simulink model "force_control_inner_loop"  (R2023a)
settings: Solver=VariableStepAuto  StartTime=0.0  StopTime=4  RelTol=1e-3
undefined symbols (not defined in the file): dqi, fd, invMd, K, KD, KF, KI, KP, Md, qi, robot, xr
settings Model: Creator=franc  LastModifiedBy=franc

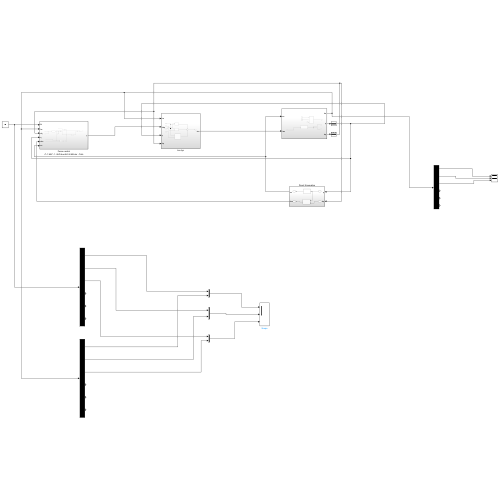
[thumbnail: Simulink's stored preview of the top-level diagram]
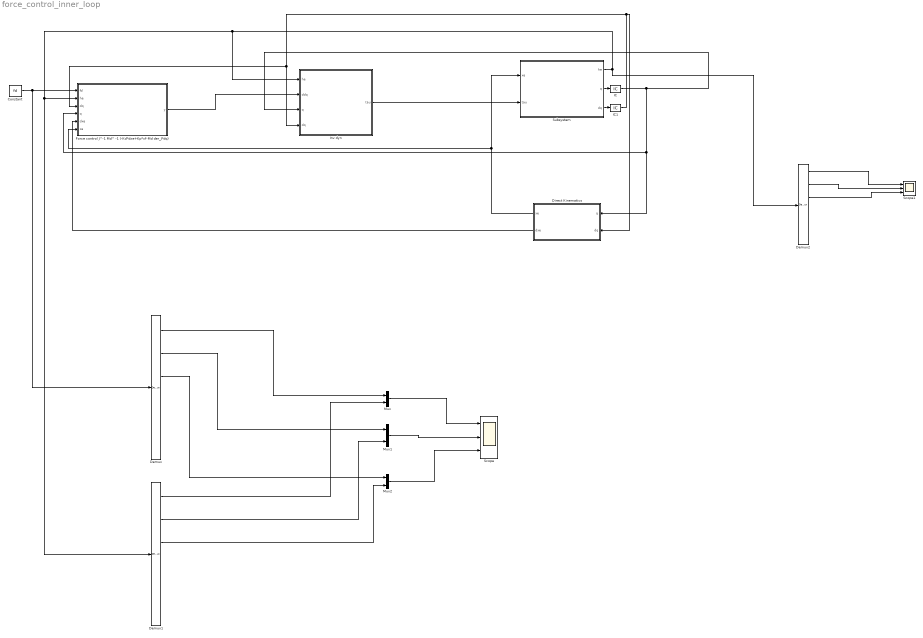
== system force_control_inner_loop ==
  Constant : Constant  Value=fd
  Demux : Demux  Outputs=6
  Demux1 : Demux  Outputs=6
  Demux2 : Demux  Outputs=6
  Direct Kinematics : Subsystem
  Force control J^-1 Md^ -1 (-Kd*dxe+Kp*xf-Md der_J*dq) : Subsystem
  IC : InitialCondition  Value=[0 0 0]
  IC1 : InitialCondition  Value=[0 0 0]
  Inv dyn : Subsystem
  Mux : Mux  Inputs=2
  Mux1 : Mux  Inputs=2
  Mux2 : Mux  Inputs=2
  Scope : Scope  NumInputPorts=3
  Scope1 : Scope  NumInputPorts=3
  Subsystem : Subsystem
  wires:
  Inv dyn/1(tau) -> Subsystem/2(tau)
  Subsystem/2(q) -> IC/1
  Subsystem/3(dq) -> IC1/1
  Direct Kinematics/1(xe) -> Subsystem/1(xe), Force control J^-1 Md^ -1 (-Kd*dxe+Kp*xf-Md der_J*dq)/6(xe)
  Direct Kinematics/2(dxe) -> Force control J^-1 Md^ -1 (-Kd*dxe+Kp*xf-Md der_J*dq)/5(dxe)
  Subsystem/1(he) -> Demux2/1, Inv dyn/1(he), Demux1/1, Force control J^-1 Md^ -1 (-Kd*dxe+Kp*xf-Md der_J*dq)/2(he)
  Force control J^-1 Md^ -1 (-Kd*dxe+Kp*xf-Md der_J*dq)/1(y) -> Inv dyn/2(ddq)
  Constant/1 -> Force control J^-1 Md^ -1 (-Kd*dxe+Kp*xf-Md der_J*dq)/1(fd), Demux/1
  Demux/1 -> Mux/1
  Demux/2 -> Mux1/1
  Demux/3 -> Mux2/1
  Demux1/1 -> Mux/2
  Demux1/2 -> Mux1/2
  Demux1/3 -> Mux2/2
  Mux/1 -> Scope/1
  Mux1/1 -> Scope/2
  Mux2/1 -> Scope/3
  IC/1 -> Force control J^-1 Md^ -1 (-Kd*dxe+Kp*xf-Md der_J*dq)/4(q), Direct Kinematics/1(q), Inv dyn/3(q)
  IC1/1 -> Force control J^-1 Md^ -1 (-Kd*dxe+Kp*xf-Md der_J*dq)/3(dq), Inv dyn/4(dq), Direct Kinematics/2(dq)
  Demux2/2 -> Scope1/2
  Demux2/1 -> Scope1/1
  Demux2/3 -> Scope1/3

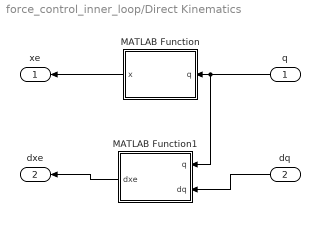
== system force_control_inner_loop/Direct Kinematics ==
  q : Inport
  dq : Inport  Port=2
  MATLAB Function : MATLAB Function  TreatAsAtomicUnit=on
  MATLAB Function1 : MATLAB Function  TreatAsAtomicUnit=on
  xe : Outport
  dxe : Outport  Port=2
  wires:
  dq/1 -> MATLAB Function1/2(dq)
  MATLAB Function1/1(dxe) -> dxe/1
  MATLAB Function/1(x) -> xe/1
  q/1 -> MATLAB Function/1(q), MATLAB Function1/1(q)

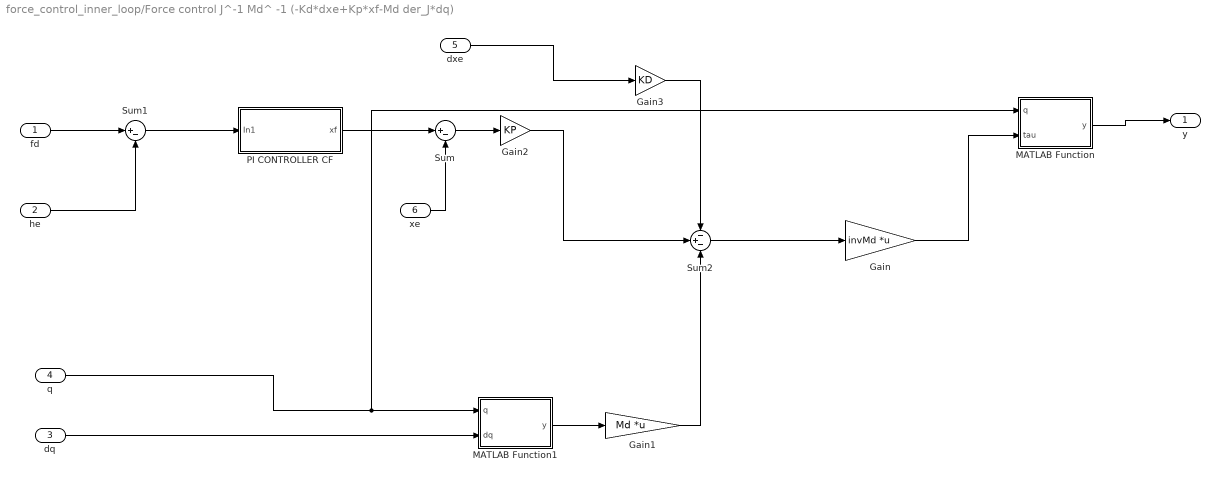
== system force_control_inner_loop/Force control J^-1 Md^ -1 (-Kd*dxe+Kp*xf-Md der_J*dq) ==
  fd : Inport
  he : Inport  Port=2
  dq : Inport  Port=3
  q : Inport  Port=4
  dxe : Inport  Port=5
  xe : Inport  Port=6
  Gain : Gain  Gain=invMd  Multiplication=Matrix(K*u)
  Gain1 : Gain  Gain=Md  Multiplication=Matrix(K*u)
  Gain2 : Gain  Gain=KP
  Gain3 : Gain  Gain=KD
  MATLAB Function : MATLAB Function  TreatAsAtomicUnit=on
  MATLAB Function1 : MATLAB Function  TreatAsAtomicUnit=on
  PI CONTROLLER CF : Subsystem
  Sum : Sum  Inputs=|+-
  Sum1 : Sum  Inputs=|+-
  Sum2 : Sum  Inputs=-+-
  y : Outport
  wires:
  fd/1 -> Sum1/1
  Sum1/1 -> PI CONTROLLER CF/1(In1)
  he/1 -> Sum1/2
  MATLAB Function/1(y) -> y/1
  Gain/1 -> MATLAB Function/2(tau)
  Sum2/1 -> Gain/1
  MATLAB Function1/1(y) -> Gain1/1
  Gain1/1 -> Sum2/3
  dq/1 -> MATLAB Function1/2(dq)
  q/1 -> MATLAB Function/1(q), MATLAB Function1/1(q)
  Gain2/1 -> Sum2/2
  dxe/1 -> Gain3/1
  Gain3/1 -> Sum2/1
  Sum/1 -> Gain2/1
  PI CONTROLLER CF/1(xf) -> Sum/1
  xe/1 -> Sum/2

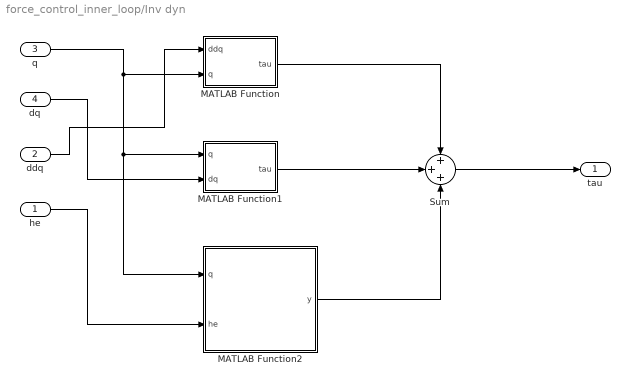
== system force_control_inner_loop/Inv dyn ==
  he : Inport
  ddq : Inport  Port=2
  q : Inport  Port=3
  dq : Inport  Port=4
  MATLAB Function : MATLAB Function  TreatAsAtomicUnit=on
  MATLAB Function1 : MATLAB Function  TreatAsAtomicUnit=on
  MATLAB Function2 : MATLAB Function  TreatAsAtomicUnit=on
  Sum : Sum  Inputs=+++
  tau : Outport
  wires:
  Sum/1 -> tau/1
  MATLAB Function1/1(tau) -> Sum/2
  MATLAB Function/1(tau) -> Sum/1
  MATLAB Function2/1(y) -> Sum/3
  q/1 -> MATLAB Function/2(q), MATLAB Function2/1(q), MATLAB Function1/1(q)
  dq/1 -> MATLAB Function1/2(dq)
  he/1 -> MATLAB Function2/2(he)
  ddq/1 -> MATLAB Function/1(ddq)

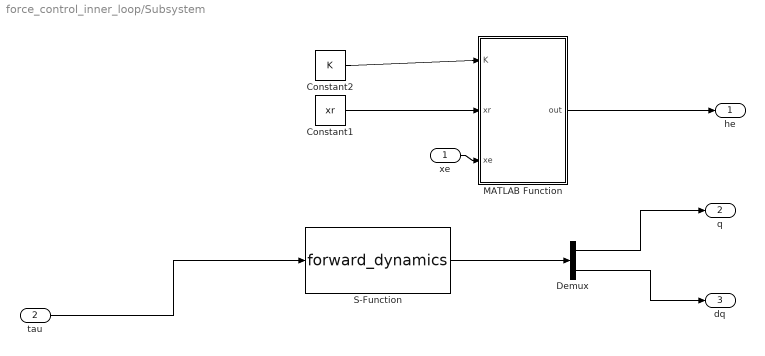
== system force_control_inner_loop/Subsystem ==
  xe : Inport
  tau : Inport  Port=2
  Constant1 : Constant  Value=xr
  Constant2 : Constant  Value=K
  Demux : Demux  Outputs=2
  MATLAB Function : MATLAB Function  TreatAsAtomicUnit=on
  S-Function : S-Function  FunctionName=forward_dynamics  Parameters=robot,qi,dqi  SFunctionDeploymentMode=off  EnableBusSupport=off
  he : Outport
  q : Outport  Port=2
  dq : Outport  Port=3
  wires:
  S-Function/1 -> Demux/1
  Constant2/1 -> MATLAB Function/1(K)
  Demux/1 -> q/1
  Constant1/1 -> MATLAB Function/2(xr)
  xe/1 -> MATLAB Function/3(xe)
  MATLAB Function/1(out) -> he/1
  tau/1 -> S-Function/1
  Demux/2 -> dq/1

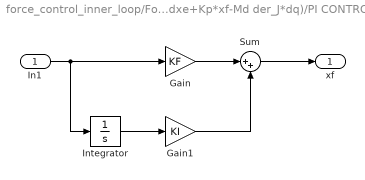
== system force_control_inner_loop/Force control J^-1 Md^ -1 (-Kd*dxe+Kp*xf-Md der_J*dq)/PI CONTROLLER CF ==
  In1 : Inport
  Gain : Gain  Gain=KF
  Gain1 : Gain  Gain=KI
  Integrator : Integrator
  Sum : Sum  Inputs=|++
  xf : Outport
  wires:
  Integrator/1 -> Gain1/1
  In1/1 -> Gain/1, Integrator/1
  Gain/1 -> Sum/1
  Gain1/1 -> Sum/2
  Sum/1 -> xf/1

== matlab function force_control_inner_loop/Force control J^-1 Md^ -1 (-Kd*dxe+Kp*xf-Md der_J*dq)/MATLAB Function ==
  data: q input; y output; tau input
function y = inv_J(q,tau)

y = get_Ja_inverse_as_9(q(1),q(2),q(3))*tau;

== matlab function force_control_inner_loop/Inv dyn/MATLAB Function ==
  data: ddq input; tau output; q input
function tau = B(ddq, q)

tau = get_B_as_7(q(1),q(3))*ddq;

== matlab function force_control_inner_loop/Inv dyn/MATLAB Function1 ==
  data: q input; tau output; dq input
function tau = n(q, dq)

tau = get_n_as_7(q(1),q(3),dq(1),dq(3));

== matlab function force_control_inner_loop/Inv dyn/MATLAB Function2 ==
  data: q input; y output; he input
function y = operational_he(q,he)

y = get_Ja_as_9(q(1),q(2),q(3))'*he;

== matlab function force_control_inner_loop/Subsystem/MATLAB Function ==
  data: K input; out output; xr input; xe input
function out = environment(K,xr, xe)
%consider the interaction only in z direction
if xe(3) > xr(3)
    out = K*(xe-xr);
else 
    out = zeros(6,1);
end

== matlab function force_control_inner_loop/Direct Kinematics/MATLAB Function ==
  data: q input; x output
function x = getK(q)

x = new_getK(q);

== matlab function force_control_inner_loop/Direct Kinematics/MATLAB Function1 ==
  data: q input; dxe output; dq input
function dxe = Ja(q,dq)

dxe = get_Ja_as_9(q(1),q(2),q(3))*dq;

== matlab function force_control_inner_loop/Force control J^-1 Md^ -1 (-Kd*dxe+Kp*xf-Md der_J*dq)/MATLAB Function1 ==
  data: q input; y output; dq input
function y = der_J(q,dq)

y = get_derivative_Ja_as_9(q(1),q(2),q(3),dq(1),dq(2),dq(3))*dq;
